simulink model "DifferetialDrive_Traj"  (R2025b)
settings: Solver=VariableStepAuto  StartTime=0.0  StopTime=50  RelTol=1e-3
values from neighbouring files (symbols this model uses):
  Kp_L = 1    [DifferentialDrive_MotorControl.m]
  Kp_theta = 1    [DifferentialDrive_MotorControl.m]
  MoveTime = 5    [DifferentialDrive_MotorControl.m]
  Ts = 0.1    [DifferentialDrive_MotorControl.m]
  Ts_vel = 1/200    (= 0.005)    [DifferentialDrive_MotorControl.m]
libraries: robotmobilelib x1, simulink x1
settings Model: Creator=ttsao  LastModifiedBy=ssw71

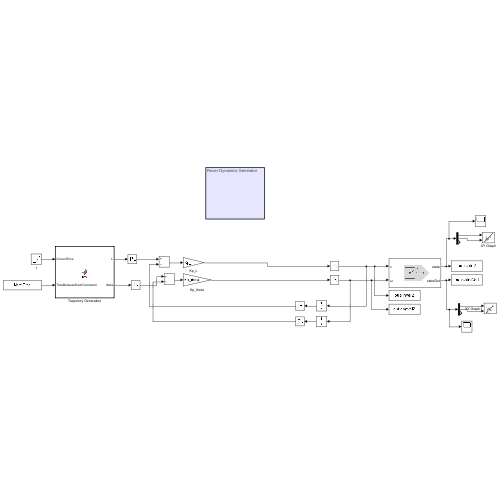
[thumbnail: Simulink's stored preview of the top-level diagram]
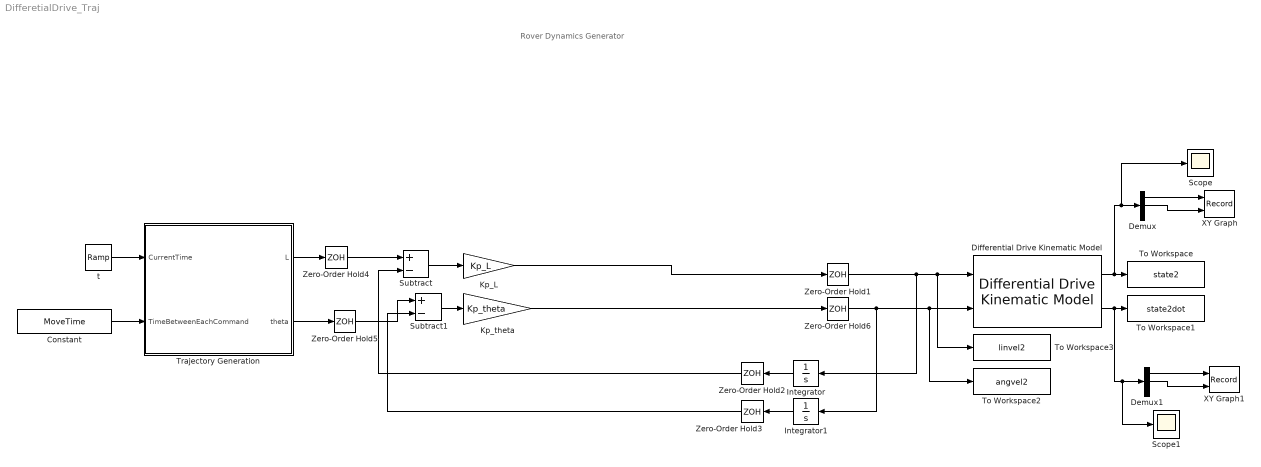
== system DifferetialDrive_Traj ==
  note: Rover Dynamics Generator
  Constant : Constant  Value=MoveTime
  Demux : Demux  Outputs=3
  Demux1 : Demux  Outputs=3
  Differential Drive Kinematic Model : robotmobilelib/Differential Drive Kinematic Model  VehicleInputs=Vehicle Speed & Heading Angular Velocity  WheelRadius=rr  WheelSpeedRange=[-inf inf]  TrackWidth=dd  InitialState=[0; 0; 0]  SimulateUsing=Interpreted execution
  Integrator : Integrator
  Integrator1 : Integrator
  Kp_L : Gain  Gain=Kp_L
  Kp_theta : Gain  Gain=Kp_theta
  Scope : Scope
      settings: ActiveDisplayYMinimum=4.9828684794438871  ActiveDisplayYMaximum=5.0012845507309391
  Scope1 : Scope
      settings: ActiveDisplayYMinimum=-1  ActiveDisplayYMaximum=1  DataLoggingVariableName=ScopeData2
  Subtract : Sum  Inputs=+-
  Subtract1 : Sum  Inputs=+-
  To Workspace : ToWorkspace  VariableName=state2  SaveFormat=Timeseries  SampleTime=-1
  To Workspace1 : ToWorkspace  VariableName=state2dot  SaveFormat=Timeseries  SampleTime=-1
  To Workspace2 : ToWorkspace  VariableName=angvel2  SaveFormat=Timeseries  SampleTime=-1
  To Workspace3 : ToWorkspace  VariableName=linvel2  SaveFormat=Timeseries  SampleTime=-1
  Trajectory Generation : MATLAB Function  TreatAsAtomicUnit=on
  XY Graph : Record  NumPorts=2.0  FileSettingsInternal="{\"entries\":[{\"content\":{\"excelSettings\":{\"content\":{},\"type\":\"Streamout.ExcelSettings\"},\"parquetSettings\":{\"content\":{},\"type\":\"Streamout.ParquetSettings\"}},\"type\":\"Streamout.FileSettingStorage\",\"uuid\":\"\"}],\"packageUris\":[\"http:\\/\\/schema.mathworks.com\\/mf0\\/streamout_blocks\\/R2020a\"],\"version\":\"1.0\"}"  FrameSettings=[0, 0]  Layout=[1 1]  SignalsInternal="{\"entries\":[{\"content\":{\"signals\":[{\"content\":{\"blockPath\":[],\"dimensions\":[1],\"domain\":\"\",\"lineColor\":\"#b746ff\",\"lineWidth\":2,\"plots\":[ 1 ],\"port\":1,\"sid\":[\"\"],\"signalID\":1,\"signalName\":\"Demux:1\"},\"type\":\"RecordBlkView.Signal\",\"uuid\":\"\"},{\"content\":{\"blockPath\":[],\"dimensions\":[1],\"domain\":\"\",\"lineColor\":\"#64d413\",\"lineWidth\":2,\"plots\":[ 1 ],\"port\":2,\"sid\":[\"\"],\"signalID\":2,\"signalName\":\"Demux:2\"},\"type\":\"RecordBlkView.Signal\",\"uuid\":\"\"}]},\"type\":\"RecordBlkView.InputSignals\",\"uuid\":\"\"}],\"packageUris\":[\"http:\\/\\/schema.mathworks.com\\/mf0\\/streamout_blocks\\/R2020a\"],\"version\":\"1.0\"}"  VisualizationBindings="{\"xyplotplugin\":{\"info\":[{\"series\":[{\"bindingParametersList\":[{\"parameter\":\"X-Axis\",\"signalID\":1,\"signalName\":\"Demux:1\"},{\"parameter\":\"Y-Axis\",\"signalID\":2,\"signalName\":\"Demux:2\"}],\"seriesID\":0}],\"subplotID\":1}]}}"  CompatibilityTag=XY
  XY Graph1 : Record  NumPorts=2.0  Filename=recording_velpcity.mldatx  FileSettingsInternal="{\"entries\":[{\"content\":{\"excelSettings\":{\"content\":{},\"type\":\"Streamout.ExcelSettings\"},\"parquetSettings\":{\"content\":{},\"type\":\"Streamout.ParquetSettings\"}},\"type\":\"Streamout.FileSettingStorage\",\"uuid\":\"\"}],\"packageUris\":[\"http:\\/\\/schema.mathworks.com\\/mf0\\/streamout_blocks\\/R2020a\"],\"version\":\"1.0\"}"  FrameSettings=[0, 0]  Layout=[1 1]  SignalsInternal="{\"entries\":[{\"content\":{\"signals\":[{\"content\":{\"blockPath\":[],\"dimensions\":[1],\"domain\":\"\",\"lineColor\":\"#a2142f\",\"plots\":[ 1 ],\"port\":1,\"sid\":[\"\"],\"signalID\":1,\"signalName\":\"Demux1:1\"},\"type\":\"RecordBlkView.Signal\",\"uuid\":\"\"},{\"content\":{\"blockPath\":[],\"dimensions\":[1],\"domain\":\"\",\"lineColor\":\"#139fff\",\"plots\":[ 1 ],\"port\":2,\"sid\":[\"\"],\"signalID\":2,\"signalName\":\"Demux1:2\"},\"type\":\"RecordBlkView.Signal\",\"uuid\":\"\"}]},\"type\":\"RecordBlkView.InputSignals\",\"uuid\":\"\"}],\"packageUris\":[\"http:\\/\\/schema.mathworks.com\\/mf0\\/streamout_blocks\\/R2020a\"],\"version\":\"1.0\"}"  VisualizationBindings="{\"xyplotplugin\":{\"info\":[{\"series\":[{\"bindingParametersList\":[{\"parameter\":\"X-Axis\",\"signalID\":1,\"signalName\":\"Demux1:1\"},{\"parameter\":\"Y-Axis\",\"signalID\":2,\"signalName\":\"Demux1:2\"}],\"seriesID\":0}],\"subplotID\":1}]}}"  CompatibilityTag=XY
  Zero-Order Hold1 : ZeroOrderHold  SampleTime=Ts_vel
  Zero-Order Hold{2..5} (4 alike) : ZeroOrderHold  SampleTime=Ts
  Zero-Order Hold6 : ZeroOrderHold  SampleTime=Ts_vel
  t : simulink/Sources/Ramp  slope=1  start=0  InitialOutput=0
  wires:
  Demux/1 -> XY Graph/1
  Demux/2 -> XY Graph/2
  Differential Drive Kinematic Model/1 -> Scope/1, Demux/1, To Workspace/1
  Kp_L/1 -> Zero-Order Hold1/1
  Kp_theta/1 -> Zero-Order Hold6/1
  Subtract/1 -> Kp_L/1
  Trajectory Generation/1(L) -> Zero-Order Hold4/1
  Integrator/1 -> Zero-Order Hold2/1
  Trajectory Generation/2(theta) -> Zero-Order Hold5/1
  Integrator1/1 -> Zero-Order Hold3/1
  Subtract1/1 -> Kp_theta/1
  Zero-Order Hold2/1 -> Subtract/2
  Zero-Order Hold3/1 -> Subtract1/2
  Zero-Order Hold4/1 -> Subtract/1
  Zero-Order Hold5/1 -> Subtract1/1
  t/1 -> Trajectory Generation/1(CurrentTime)
  Constant/1 -> Trajectory Generation/2(TimeBetweenEachCommand)
  Demux1/1 -> XY Graph1/1
  Differential Drive Kinematic Model/2 -> Scope1/1, Demux1/1, To Workspace1/1
  Demux1/2 -> XY Graph1/2
  Zero-Order Hold1/1 -> To Workspace3/1, Differential Drive Kinematic Model/1, Integrator/1
  Zero-Order Hold6/1 -> Integrator1/1, To Workspace2/1, Differential Drive Kinematic Model/2

== matlab function DifferetialDrive_Traj/Trajectory Generation ==
  data: L output; theta output; CurrentTime input; TimeBetweenEachCommand input
function [L, theta]= fcn(CurrentTime, TimeBetweenEachCommand)

L_array     = [0 5 10 ];
Theta_array = [0 0  0 ];
L_array     = [0 5 10   10   15 ];
Theta_array = [0 0  0 pi/2 pi/2 ];
L_array     = [0 5 10   10   15   15+10*pi/4   ];
Theta_array = [0 0  0 pi/2 pi/2           pi   ];
%L_array     = [0 5 10   10   15   15+10*pi/4     10*pi/4+20  10*pi/4+20   10*pi/4+30];
%Theta_array = [0 0  0 pi/2 pi/2           pi             pi    1.5*pi       1.5*pi ];


index = floor(CurrentTime/TimeBetweenEachCommand) + 1;
if index>length(L_array)
    index = length(L_array);
end
L = L_array(index);
theta = Theta_array(index);
